simulink model "simulacion_tres_tanques_loop"  (R2015b)
settings: Solver=ode45  StartTime=0.0  StopTime=10.0  RelTol=1e-3
settings Model: Creator=nico  LastModifiedBy=nico
settings DataIOCC: SaveFormat=StructureWithTime
settings HardwareCC: ProdWordSize=32  ProdHWDeviceType=Specified

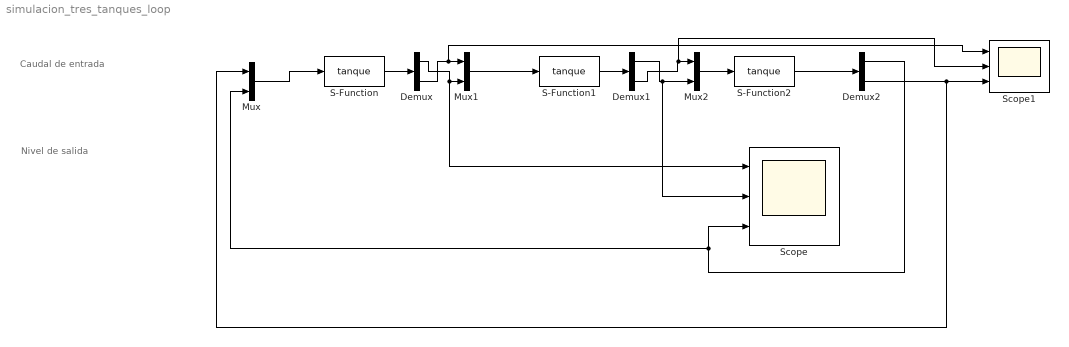
== system simulacion_tres_tanques_loop ==
  note: Nivel de salida
  note: Caudal de entrada
  Demux : Demux  Outputs=2
  Demux1 : Demux  Outputs=2
  Demux2 : Demux  Outputs=2
  Mux : Mux  Inputs=2
  Mux1 : Mux  Inputs=2
  Mux2 : Mux  Inputs=2
  S-Function : S-Function  FunctionName=tanque  Parameters=1 8 1 2  SFunctionDeploymentMode=off  EnableBusSupport=off
  S-Function1 : S-Function  FunctionName=tanque  Parameters=1 8 1 7  SFunctionDeploymentMode=off  EnableBusSupport=off
  S-Function2 : S-Function  FunctionName=tanque  Parameters=1 8 1 3  SFunctionDeploymentMode=off  EnableBusSupport=off
  Scope : Scope  NumInputPorts=3
  Scope1 : Scope  NumInputPorts=3
  wires:
  Demux2/1 -> Mux/2, Scope/3
  Mux/1 -> S-Function/1
  Demux2/2 -> Mux/1, Scope1/3
  S-Function/1 -> Demux/1
  Demux/2 -> Scope1/1, Mux1/1
  Demux/1 -> Scope/1, Mux1/2
  Mux1/1 -> S-Function1/1
  Mux2/1 -> S-Function2/1
  S-Function1/1 -> Demux1/1
  Demux1/1 -> Scope/2, Mux2/2
  Demux1/2 -> Scope1/2, Mux2/1
  S-Function2/1 -> Demux2/1
